simulink model "room_heating_0508"  (R2017b)
settings: Solver=ode4  StartTime=0.0  StopTime=3600  FixedStep=0.01  RelTol=1e-3
values from neighbouring files (symbols this model uses):
  c_Wasser = 4184.0    [Data_Dictionary_room_heating.sldd]
  I_Heizelement = 60000.0    [Data_Dictionary_room_heating.sldd]
  ks = 0.99717641281663061    [Data_Dictionary_room_heating.sldd]
  m_Kessel = 150.0    [Data_Dictionary_room_heating.sldd]
  R_Oberflaeche = 6.2099999999999992E-5    [Data_Dictionary_room_heating.sldd]
  Ts = 46.675708884069117    [Data_Dictionary_room_heating.sldd]
libraries: simulink x2
settings Model: DataDictionary=Data_Dictionary_room_heating.sldd  Creator=y03li  LastModifiedBy=y03li
settings OptimizationCC: LocalBlockOutputs=off
settings RTWCC: SystemTargetFile=TwinCAT.tlc  GenCodeOnly=on  MakeCommand=make_tct  TemplateMakefile=tct_msbuild.tmf  Description=TwinCAT Target  GenerateReport=on  TargetLang=C++
settings STFCustomTargetCC: TargetLangStandard=C++03 (ISO)  CompOptLevelCompliant=on  MATLABClassNameForMDSCustomization=Simulink.SoftwareTarget.TargetSpecificTriggerConfigurationBase  SystemTargetFile=TwinCAT.tlc

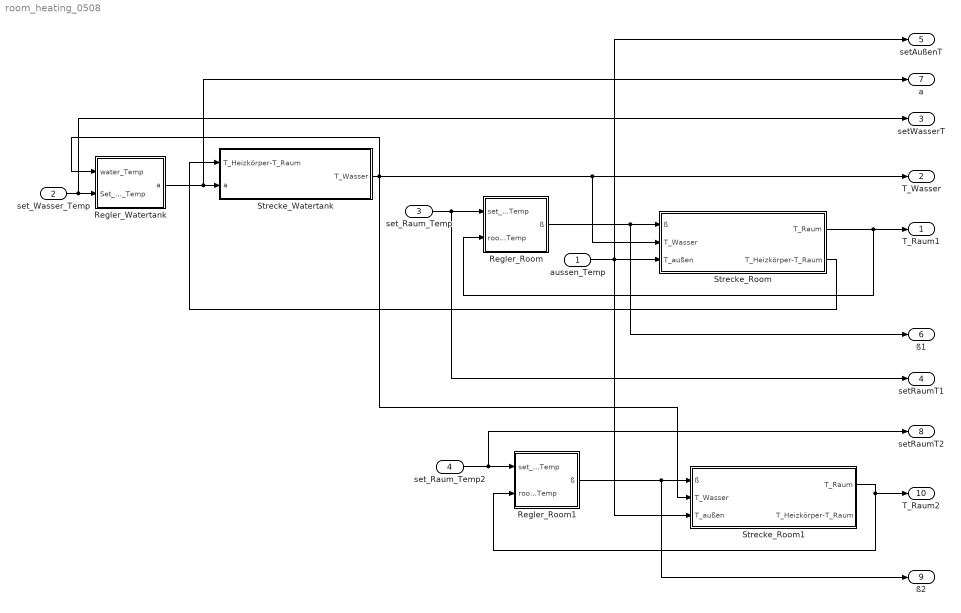
== system room_heating_0508 ==
  aussen_Temp : Inport
  set_Wasser_Temp : Inport  Port=2
  set_Raum_Temp : Inport  Port=3
  set_Raum_Temp2 : Inport  Port=4
  Regler_Room : Subsystem
  Regler_Room1 : Subsystem
  Regler_Watertank : Subsystem
  Strecke_Room : Subsystem
  Strecke_Room1 : Subsystem
  Strecke_Watertank : Subsystem
  T_Raum1 : Outport
  T_Wasser : Outport  Port=2
  setWasserT : Outport  Port=3
  setRaumT1 : Outport  Port=4
  setAußenT : Outport  Port=5
  ß1 : Outport  Port=6
  a : Outport  Port=7
  setRaumT2 : Outport  Port=8
  ß2 : Outport  Port=9
  T_Raum2 : Outport  Port=10
  wires:
  Strecke_Room/1(T_Raum) -> Regler_Room/2(room_Temp), T_Raum1/1
  Strecke_Watertank/1(T_Wasser) -> Strecke_Room/2(T_Wasser), T_Wasser/1, Regler_Watertank/1(water_Temp), Strecke_Room1/2(T_Wasser)
  Strecke_Room/2(T_Heizkörper-T_Raum) -> Strecke_Watertank/1(T_Heizkörper-T_Raum)
  Regler_Watertank/1(a) -> a/1, Strecke_Watertank/2(a)
  Regler_Room/1(ß) -> ß1/1, Strecke_Room/1(ß)
  set_Raum_Temp/1 -> Regler_Room/1(set_room_Temp), setRaumT1/1
  set_Wasser_Temp/1 -> setWasserT/1, Regler_Watertank/2(Set_water_Temp)
  set_Raum_Temp2/1 -> setRaumT2/1, Regler_Room1/1(set_room_Temp)
  Regler_Room1/1(ß) -> ß2/1, Strecke_Room1/1(ß)
  Strecke_Room1/1(T_Raum) -> T_Raum2/1, Regler_Room1/2(room_Temp)
  aussen_Temp/1 -> Strecke_Room1/3(T_außen), setAußenT/1, Strecke_Room/3(T_außen)

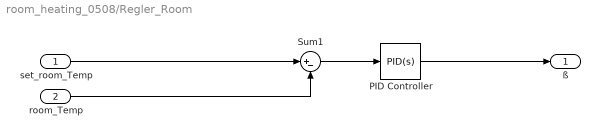
== system room_heating_0508/Regler_Room ==
  set_room_Temp : Inport
  room_Temp : Inport  Port=2
  PID Controller : simulink/Continuous/PID Controller  Controller=PID  TimeDomain=Continuous-time  SampleTime=-1  IntegratorMethod=Forward Euler  FilterMethod=Forward Euler  Form=Parallel  UseFilter=on  ControllerParametersSource=internal  P=0.5/(ks*60)  I=0.5/(ks*60)/(0.8*Ts)  D=0  N=100  InitialConditionSource=internal  InitialConditionForIntegrator=0  InitialConditionForFilter=0  ExternalReset=none  LimitOutput=off  UpperSaturationLimit=1  LowerSaturationLimit=0  LinearizeAsGain=on  AntiWindupMode=none  Kb=1  TrackingMode=off  Kt=1  PParamMin=[]  PParamMax=[]  IParamMin=[]  IParamMax=[]  DParamMin=[]  DParamMax=[]  NParamMin=[]  NParamMax=[]  KbParamMin=[]  KbParamMax=[]  KtParamMin=[]  KtParamMax=[]  POutMin=[]  POutMax=[]  IOutMin=[]  IOutMax=[]  DOutMin=[]  DOutMax=[]  NOutMin=[]  NOutMax=[]  KbOutMin=[]  KbOutMax=[]  KtOutMin=[]  KtOutMax=[]  IntegratorOutMin=[]  IntegratorOutMax=[]  FilterOutMin=[]  FilterOutMax=[]  SumOutMin=[]  SumOutMax=[]  SumI1OutMin=[]  SumI1OutMax=[]  SumI2OutMin=[]  SumI2OutMax=[]  SumI3OutMin=[]  SumI3OutMax=[]  SumDOutMin=[]  SumDOutMax=[]  SaturationOutMin=[]  SaturationOutMax=[]  IntegratorContinuousStateAttributes=''  IntegratorStateMustResolveToSignalObject=off  IntegratorRTWStateStorageClass=Auto  FilterContinuousStateAttributes=''  FilterStateMustResolveToSignalObject=off  FilterRTWStateStorageClass=Auto  DifferentiatorICPrevScaledInput=0  DifferentiatorOutMin=[]  DifferentiatorOutMax=[]  InitialConditionSetting=State (most efficient)  FilterDiffOutCoefMin=[]  FilterDiffOutCoefMax=[]  SumDenOutMin=[]  SumDenOutMax=[]  SumNumOutMin=[]  SumNumOutMax=[]  ReciprocalOutMin=[]  ReciprocalOutMax=[]  DivideOutMin=[]  DivideOutMax=[]  TunerSelectOption=Transfer Function Based (PID Tuner App)
  Sum1 : Sum  Inputs=|+-
  ß : Outport
  wires:
  PID Controller/1 -> ß/1
  set_room_Temp/1 -> Sum1/1
  Sum1/1 -> PID Controller/1
  room_Temp/1 -> Sum1/2

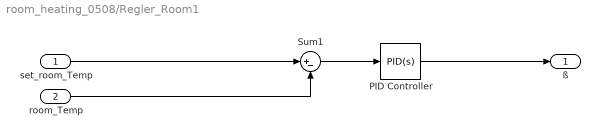
== system room_heating_0508/Regler_Room1 ==
  set_room_Temp : Inport
  room_Temp : Inport  Port=2
  PID Controller : simulink/Continuous/PID Controller  Controller=PID  TimeDomain=Continuous-time  SampleTime=-1  IntegratorMethod=Forward Euler  FilterMethod=Forward Euler  Form=Parallel  UseFilter=on  ControllerParametersSource=internal  P=0.5/(ks*60)  I=0.5/(ks*60)/(0.8*Ts)  D=0  N=100  InitialConditionSource=internal  InitialConditionForIntegrator=0  InitialConditionForFilter=0  ExternalReset=none  LimitOutput=off  UpperSaturationLimit=1  LowerSaturationLimit=0  LinearizeAsGain=on  AntiWindupMode=none  Kb=1  TrackingMode=off  Kt=1  PParamMin=[]  PParamMax=[]  IParamMin=[]  IParamMax=[]  DParamMin=[]  DParamMax=[]  NParamMin=[]  NParamMax=[]  KbParamMin=[]  KbParamMax=[]  KtParamMin=[]  KtParamMax=[]  POutMin=[]  POutMax=[]  IOutMin=[]  IOutMax=[]  DOutMin=[]  DOutMax=[]  NOutMin=[]  NOutMax=[]  KbOutMin=[]  KbOutMax=[]  KtOutMin=[]  KtOutMax=[]  IntegratorOutMin=[]  IntegratorOutMax=[]  FilterOutMin=[]  FilterOutMax=[]  SumOutMin=[]  SumOutMax=[]  SumI1OutMin=[]  SumI1OutMax=[]  SumI2OutMin=[]  SumI2OutMax=[]  SumI3OutMin=[]  SumI3OutMax=[]  SumDOutMin=[]  SumDOutMax=[]  SaturationOutMin=[]  SaturationOutMax=[]  IntegratorContinuousStateAttributes=''  IntegratorStateMustResolveToSignalObject=off  IntegratorRTWStateStorageClass=Auto  FilterContinuousStateAttributes=''  FilterStateMustResolveToSignalObject=off  FilterRTWStateStorageClass=Auto  DifferentiatorICPrevScaledInput=0  DifferentiatorOutMin=[]  DifferentiatorOutMax=[]  InitialConditionSetting=State (most efficient)  FilterDiffOutCoefMin=[]  FilterDiffOutCoefMax=[]  SumDenOutMin=[]  SumDenOutMax=[]  SumNumOutMin=[]  SumNumOutMax=[]  ReciprocalOutMin=[]  ReciprocalOutMax=[]  DivideOutMin=[]  DivideOutMax=[]  TunerSelectOption=Transfer Function Based (PID Tuner App)
  Sum1 : Sum  Inputs=|+-
  ß : Outport
  wires:
  PID Controller/1 -> ß/1
  set_room_Temp/1 -> Sum1/1
  Sum1/1 -> PID Controller/1
  room_Temp/1 -> Sum1/2

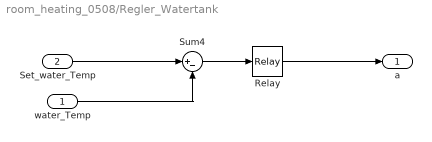
== system room_heating_0508/Regler_Watertank ==
  water_Temp : Inport
  Set_water_Temp : Inport  Port=2
  Relay : Relay  OnSwitchValue=0.5  OffSwitchValue=-0.5
  Sum4 : Sum  Inputs=|+-
  a : Outport
  wires:
  Relay/1 -> a/1
  Sum4/1 -> Relay/1
  Set_water_Temp/1 -> Sum4/1
  water_Temp/1 -> Sum4/2

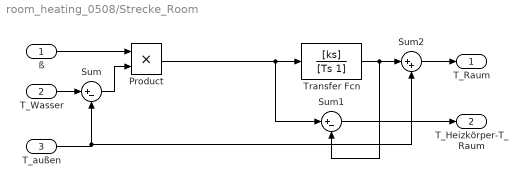
== system room_heating_0508/Strecke_Room ==
  ß : Inport
  T_Wasser : Inport  Port=2
  T_außen : Inport  Port=3
  Product : Product
  Sum : Sum  Inputs=|+-
  Sum1 : Sum  Inputs=|+-
  Sum2 : Sum  Inputs=|++
  Transfer Fcn : TransferFcn  Numerator=[ks]  Denominator=[Ts 1]
  T_Raum : Outport
  T_Heizkörper-T_Raum : Outport  Port=2
  wires:
  ß/1 -> Product/1
  Transfer Fcn/1 -> Sum1/2, Sum2/1
  Sum2/1 -> T_Raum/1
  Sum/1 -> Product/2
  Product/1 -> Transfer Fcn/1, Sum1/1
  T_Wasser/1 -> Sum/1
  T_außen/1 -> Sum2/2, Sum/2
  Sum1/1 -> T_Heizkörper-T_Raum/1

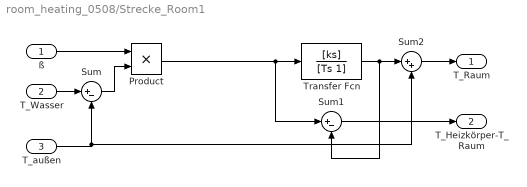
== system room_heating_0508/Strecke_Room1 ==
  ß : Inport
  T_Wasser : Inport  Port=2
  T_außen : Inport  Port=3
  Product : Product
  Sum : Sum  Inputs=|+-
  Sum1 : Sum  Inputs=|+-
  Sum2 : Sum  Inputs=|++
  Transfer Fcn : TransferFcn  Numerator=[ks]  Denominator=[Ts 1]
  T_Raum : Outport
  T_Heizkörper-T_Raum : Outport  Port=2
  wires:
  ß/1 -> Product/1
  Transfer Fcn/1 -> Sum1/2, Sum2/1
  Sum2/1 -> T_Raum/1
  Sum/1 -> Product/2
  Product/1 -> Transfer Fcn/1, Sum1/1
  T_Wasser/1 -> Sum/1
  T_außen/1 -> Sum2/2, Sum/2
  Sum1/1 -> T_Heizkörper-T_Raum/1

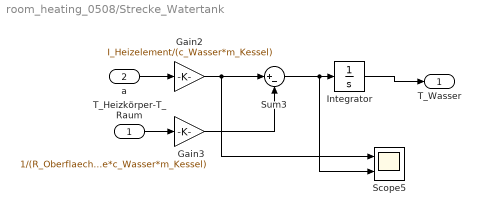
== system room_heating_0508/Strecke_Watertank ==
  T_Heizkörper-T_Raum : Inport
  a : Inport  Port=2
  Gain2 : Gain  Gain=I_Heizelement/(c_Wasser*m_Kessel)
  Gain3 : Gain  Gain=1/(R_Oberflaeche*c_Wasser*m_Kessel)
  Integrator : Integrator  InitialCondition=20
  Scope5 : Scope  NumInputPorts=2
  Sum3 : Sum  Inputs=|+-
  T_Wasser : Outport
  wires:
  Gain2/1 -> Scope5/1, Sum3/1
  a/1 -> Gain2/1
  Integrator/1 -> T_Wasser/1
  Gain3/1 -> Sum3/2
  Sum3/1 -> Scope5/2, Integrator/1
  T_Heizkörper-T_Raum/1 -> Gain3/1
